simulink model "s_rotpen_bal"  (R2020a)
settings: Solver=ode1  StartTime=0.0  StopTime=10  FixedStep=0.002  RelTol=1e-3  EnableMultiTasking=on
undefined symbols (not defined in the file or in its folder): A, a_max, B, C, D, K, wcf_1, wcf_2
libraries: simulink_extras x3
settings Model: ExtModeTrigDuration=10000  Creator=MLevis  LastModifiedBy=sinow
settings SolverCC: PositivePriorityOrder=on
settings DataIOCC: LimitDataPoints=on  SaveFormat=Array  SignalLoggingSaveFormat=ModelDataLogs  ReturnWorkspaceOutputs=off
settings OptimizationCC: BooleanDataType=off  OptimizeBlockIOStorage=off  BufferReuse=off  GlobalBufferReuse=off  ExpressionFolding=off  ExpressionDepthLimit=2147483647  LocalBlockOutputs=off  InitFltsAndDblsToZero=on  LifeSpan=inf  OptimizeDataStoreBuffers=off  BusAssignmentInplaceUpdate=off
settings DebuggingCC: SaveWithParameterizedLinksMsg=none  UnderspecifiedInitializationDetection=Classic  MergeDetectMultiDrivingBlocksExec=none  SignalResolutionControl=TryResolveAllWithWarning  MultiTaskDSMMsg=warning  MultiTaskCondExecSysMsg=none  FcnCallInpInsideContextMsg=warning  StateNameClashWarn=warning  SFUnexpectedBacktrackingDiag=warning  SFNoUnconditionalDefaultTransitionDiag=warning  SFExecutionAtInitializationDiag=none  ArithmeticOperatorsInVariantConditions=warning
settings HardwareCC: ProdBitPerPointer=32  ProdBitPerSizeT=32  ProdBitPerPtrDiffT=32  ProdLargestAtomicFloat=None  ProdIntDivRoundTo=Undefined  ProdEndianess=Unspecified  ProdWordSize=32  ProdHWDeviceType=32-bit Generic  TargetHWDeviceType=32-bit Generic
settings ModelReferenceCC: PropagateSignalLabelsOutOfModel=off
settings SFSimCC: CustomCodeUndefinedFunction=UseInterfaceOnly
settings RTWCC: Description=Quarc Win32 Target  SystemTargetFile=quarc_windows.tlc  TemplateMakefile=quarc_default_tmf
settings CodeAppCC: StateflowObjectComments=on
settings STFCustomTargetCC: TargetFcnLib=ansi_tfl_tmw.mat  TargetPreCompLibLocation=C:\PROGRA~3\QUARC\lib\2018b\windows\release  CPPClassGenCompliant=on  GRTInterface=on  SystemTargetFile=quarc_windows.tlc
settings GRTTargetCC: TargetFcnLib=ansi_tfl_tmw.mat  TargetPreCompLibLocation=C:\PROGRA~3\QUARC\lib\2018b\windows\release  TargetLangStandard=C89/C90 (ANSI)  ParMdlRefBuildCompliant=off  CompOptLevelCompliant=off  ConcurrentExecutionCompliant=off  CombineOutputUpdateFcns=off  MatFileLogging=off  GRTInterface=on  UseToolchainInfoCompliant=off  ExtMode=on  ExtModeMexFile=quarc_comm
settings ConfigComp: CovMetricSettings=dw  CovHtmlReporting=on  CovSaveCumulativeToWorkspaceVar=on  CovSaveSingleToWorkspaceVar=on

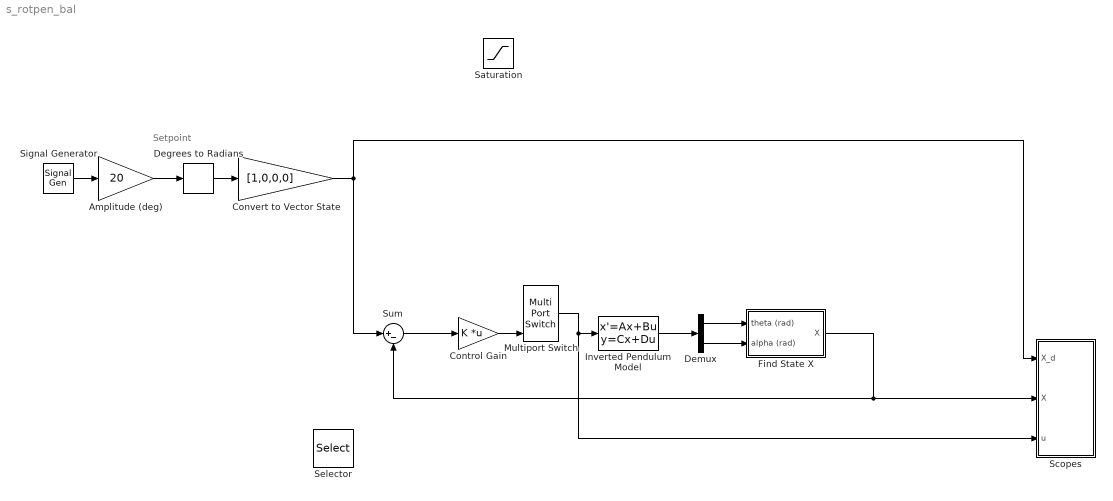
== system s_rotpen_bal ==
  note: Setpoint
  Amplitude (deg) : Gain  Gain=20  SaturateOnIntegerOverflow=on  OutDataTypeStr=Inherit: Same as input  ParamDataTypeStr=Inherit: Same as input
  Control Gain : Gain  Gain=K  Multiplication=Matrix(K*u)
  Convert to Vector State : Gain  Gain=[1,0,0,0]
  Degrees to Radians : simulink_extras/Transformations/Degrees to Radians
  Demux : Demux  Outputs=2
  Find State X : Subsystem
  Inverted Pendulum Model : StateSpace  A=A  B=B  C=C  D=D  InitialCondition=0
  Multiport Switch : MultiPortSwitch  Inputs=2
  Saturation : Saturate  UpperLimit=a_max  LowerLimit=-a_max
  Scopes : Subsystem
  Selector : Selector  NumberOfDimensions=4  InputPortWidth=3  IndexOptions=Index vector (dialog),Index vector (dialog),Index vector (dialog),Index vector (dialog)  Indices=[1 3],1,1,1  OutputSizes=1,1,1,1
  Signal Generator : SignalGenerator  WaveForm=square  Frequency=0.1
  Sum : Sum  Inputs=|+-
  wires:
  Amplitude (deg)/1 -> Degrees to Radians/1
  Signal Generator/1 -> Amplitude (deg)/1
  Degrees to Radians/1 -> Convert to Vector State/1
  Convert to Vector State/1 -> Sum/1, Scopes/1(X_d)
  Find State X/1(X) -> Sum/2, Scopes/2(X)
  Sum/1 -> Control Gain/1
  Control Gain/1 -> Multiport Switch/3
  Inverted Pendulum Model/1 -> Demux/1
  Demux/1 -> Find State X/1(theta (rad))
  Demux/2 -> Find State X/2(alpha (rad))
  Multiport Switch/1 -> Scopes/3(u), Inverted Pendulum Model/1

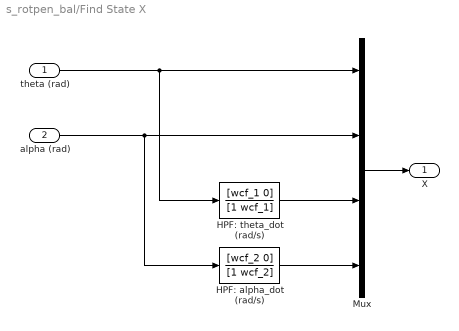
== system s_rotpen_bal/Find State X ==
  theta (rad) : Inport
  alpha (rad) : Inport  Port=2
  HPF: alpha_dot (rad/s) : TransferFcn  Numerator=[wcf_2 0]  Denominator=[1 wcf_2]
  HPF: theta_dot (rad/s) : TransferFcn  Numerator=[wcf_1 0]  Denominator=[1 wcf_1]
  Mux : Mux
  X : Outport  VectorParamsAs1DForOutWhenUnconnected=off
  wires:
  alpha (rad)/1 -> Mux/2, HPF: alpha_dot (rad/s)/1
  Mux/1 -> X/1
  theta (rad)/1 -> Mux/1, HPF: theta_dot (rad/s)/1
  HPF: theta_dot (rad/s)/1 -> Mux/3
  HPF: alpha_dot (rad/s)/1 -> Mux/4

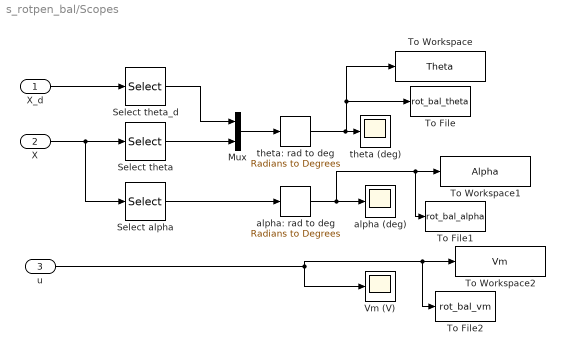
== system s_rotpen_bal/Scopes ==
  X_d : Inport
  X : Inport  Port=2
  u : Inport  Port=3
  Mux : Mux  Inputs=2
  Select alpha : Selector  InputPortWidth=4  IndexOptions=Index vector (dialog)  Indices=2  OutputSizes=[(-2)]
  Select theta : Selector  InputPortWidth=4  IndexOptions=Index vector (dialog)  Indices=1  OutputSizes=[(-2)]
  Select theta_d : Selector  InputPortWidth=4  IndexOptions=Index vector (dialog)  Indices=1  OutputSizes=[(-2)]
  To File : ToFile  Filename=rot_bal_theta  SaveFormat=Timeseries
  To File1 : ToFile  Filename=rot_bal_alpha  SaveFormat=Timeseries
  To File2 : ToFile  Filename=rot_bal_vm  SaveFormat=Timeseries
  To Workspace : ToWorkspace  VariableName=Theta  SaveFormat=Timeseries  SampleTime=-1
  To Workspace1 : ToWorkspace  VariableName=Alpha  SaveFormat=Timeseries  SampleTime=-1
  To Workspace2 : ToWorkspace  VariableName=Vm  SaveFormat=Timeseries  SampleTime=-1
  Vm (V) : Scope
  alpha (deg) : Scope
  alpha: rad to deg : simulink_extras/Transformations/Radians to Degrees
  theta (deg) : Scope
  theta: rad to deg : simulink_extras/Transformations/Radians to Degrees
  wires:
  X_d/1 -> Select theta_d/1
  Select alpha/1 -> alpha: rad to deg/1
  X/1 -> Select alpha/1, Select theta/1
  Select theta_d/1 -> Mux/1
  Select theta/1 -> Mux/2
  u/1 -> To File2/1, To Workspace2/1, Vm (V)/1
  alpha: rad to deg/1 -> To File1/1, To Workspace1/1, alpha (deg)/1
  Mux/1 -> theta: rad to deg/1
  theta: rad to deg/1 -> To File/1, To Workspace/1, theta (deg)/1
